simulink library "mylib"  (R2020a)
settings: Solver=VariableStepAuto  StartTime=0.0  StopTime=10.0  RelTol=1e-3
undefined symbols (not defined in the file): d_du_max_pu, dir_to_bus1, dir_to_bus_0L, dir_to_bus_2, dir_to_line1, dir_to_line_0L, dir_to_line_2, du_max_pu, du_ph_max_pu, Fi_0, Fi_T_H, Fi_T_L, Fi_T_M, I0_calc_0L, I0_comp_H, I0_comp_L, I0_comp_M, I0_max_0L, I2_max_2, I_diff1, I_diff2, I_diff3, I_diff4, I_diff5, I_diff_to, I_hight_CT1_G, I_hight_CT2_G, I_low_CT1, I_low_CT2, I_max1, I_max2, I_max3, I_max4, I_max5, I_min_sec_CT1, I_min_sec_CT2, I_unb, Iph_max_0L, Iph_max_2, jmp_in_zone, jmp_in_zone_0L, jmp_in_zone_2, K_dop, max_min1, only_K1_0L, only_K1_2, only_K2_0L, only_K2_2, only_K3_0L, only_K3_2, P_ctl_0, PQ_Fi_ctl_0, Q_ctl_0, S_set_0, set, set1, T_fast, T_I_ctl, T_off, T_on ... (+15)
libraries: $bdroot x184, powerlib_meascontrol x97
(part 1 of 14)
settings Model: Creator=Fasedus  LastModifiedBy=Александр
settings DataIOCC: ReturnWorkspaceOutputs=off
settings DebuggingCC: ArithmeticOperatorsInVariantConditions=warning
settings SFSimCC: SimUseLocalCustomCode=off  CustomCodeUndefinedFunction=UseInterfaceOnly
settings RTWCC: RTWUseLocalCustomCode=off
settings CodeAppCC: StateflowObjectComments=on

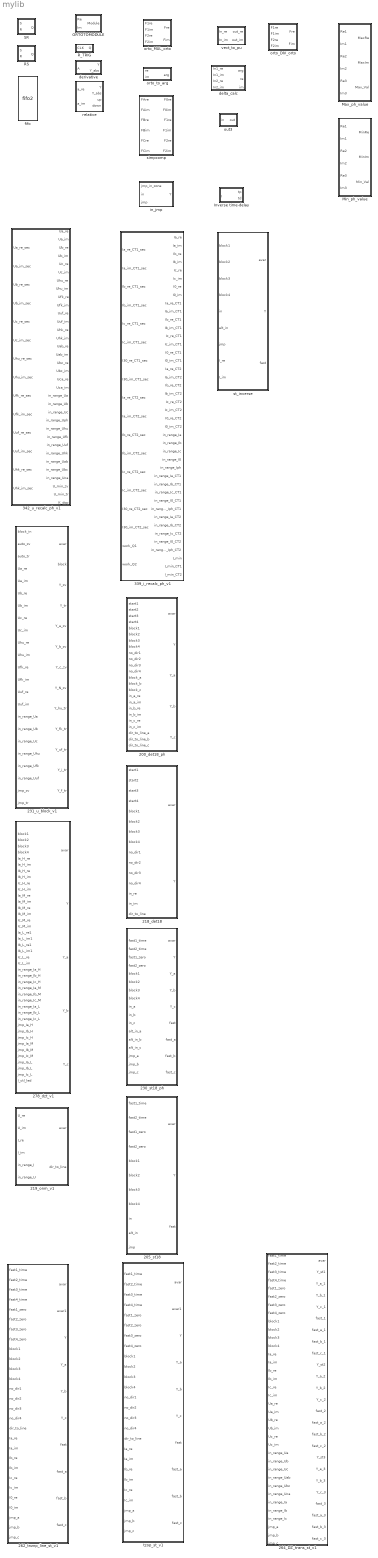
== system mylib ==
  200_det18_ph : Subsystem  mask{det=[max_min1, set1, dir_to_line1, dir_to_bus1]}
      mask prompts: det "det [max_min, set, dir_to_line, dir_to_bus]"
      mask init:
      | max_min = det(1);
      | set = det(2);
      | dir_to_line = det(3);
      | dir_to_bus = det(4);
  205_st18 : Subsystem  AncestorBlock=mylib/205_st18  mask{st18_ph=[1, 1, 1, 0, T_reset, 0, T_st_sign, T_out]}
      mask prompts: st18_ph "st18_ph [only_K1, only_K2, only_K3, jmp_in_zone, T_reset, T_fast, T_st, T_out]"
      mask init:
      | only_K1 = st18_ph(1);
      | only_K2 = st18_ph(2); 
      | only_K3 = st18_ph(3); 
      | jmp_in_zone = st18_ph(4);
      | T_reset = st18_ph(5);
      | T_fast = st18_ph(6); 
      | T_st = st18_ph(7); 
      | T_out = st18_ph(8);
  218_det18 : Subsystem  AncestorBlock=mylib/218_det18  mask{det=[0, set, 0, 0]}
      mask prompts: det "det [max_min, set, dir_to_line, dir_to_bus]"
      mask init:
      | max_min = det(1);
      | set = det(2);
      | dir_to_line = det(3);
      | dir_to_bus = det(4);
  219_onm_v1 : Subsystem  mask{onm_v1=[PQ_Fi_ctl_0, P_ctl_0, Q_ctl_0, U_dir_PQ_0,S_set_0, Fi_0]}
      mask prompts: onm_v1 "onm_v1[PQ_Fi_ctl, P_ctl, Q_ctl, U_dir_PQ,S_set, Fi]"
      mask init:
      | PQ_Fi_ctl= onm_v1(1);
      | P_ctl = onm_v1(2);
      | Q_ctl = onm_v1(3); 
      | U_dir_PQ = onm_v1(4);
      | S_set = onm_v1(5); 
      | Fi = onm_v1(6);
  230_st18_ph : Subsystem  AncestorBlock=mylib/230_st18_ph  mask{st18_ph=[1, 1, 1, 0, T_reset, T_fast, T_st, T_out]}
      mask prompts: st18_ph "st18_ph [only_K1, only_K2, only_K3, jmp_in_zone, T_reset, T_fast, T_st, T_out]"
      mask init:
      | only_K1 = st18_ph(1);
      | only_K2 = st18_ph(2); 
      | only_K3 = st18_ph(3); 
      | jmp_in_zone = st18_ph(4);
      | T_reset = st18_ph(5);
      | T_fast = st18_ph(6); 
      | T_st = st18_ph(7); 
      | T_out = st18_ph(8);
  231_u_block_v1 : Subsystem  mask{Ublock=[K_dop, du_ph_max_pu, du_max_pu, d_du_max_pu]}
      mask prompts: Ublock "Ublock [ K_dop, du_ph_max_pu,du_max_pu, d_du_max_pu]"
      mask init:
      | K_dop = Ublock(1);
      | du_ph_max_pu = Ublock(2);
      | du_max_pu = Ublock(3); 
      | d_du_max_pu = Ublock(4);
  262_tnznp_line_st_v1 : Subsystem  mask{tnznp_line=[I0_calc_0L,I0_max_0L, Iph_max_0L, dir_to_line_0L, dir_to_bus_0L, only_K1_0L, only_K2_0L, only_K3_0L, jmp_in_zone_0L, T_st_0L]}
      mask prompts: tnznp_line "tnznp_line [I0_calc, Iph_max, dir_to_line, dir_to_bus, only_K1, only_K2, only_K3, jmp_in_zone, T_st]"
      mask init:
      | I0_calc = tnznp_line(1);
      | I0_max = tnznp_line(2);
      | Iph_max = tnznp_line(3); 
      | dir_to_line = tnznp_line(4);
      | dir_to_bus = tnznp_line(5);
      | only_K1 = tnznp_line(6); 
      | only_K2 = tnznp_line(7); 
      | only_K3 = tnznp_line(8); 
      | jmp_in_zone = tnznp_line(9); 
      | T_st = tnznp_line(10);
  264_DZ_trans_st_v1 : Subsystem  mask{DZ_trans_time=[1, 2, 3], DZ_trans_Calc1=[5, 0.00151, 0.219, 1000], DZ_trans_Calc2=[0, 20000, 0, 0], DZ_trans_PolySet1=[0, 0, -10, 10, -15, 30, -20, 120, 10, 80, 20, 100], DZ_trans_PolySet2=[40, 100, 40, 70, 60, 70, 80, 40, 90, 30, 20, 30]}
      mask prompts: DZ_trans_time "[T_st1, T_st2, T_st3]"; DZ_trans_Calc1 "[arg_U_K2, R, X, U_kz_pu_r_rem ]"; DZ_trans_Calc2 "[ph_to_line, U_nom_ph, recalc_Z_ph, recalc_Z_lin]"; DZ_trans_PolySet1 "[R_1, X_1, R_2, X_2, R_3, X_3, R_4, X_4, R_5, X_5, R_6, X_6]"; DZ_trans_PolySet2 "[R_7, X_7, R_8, X_8, R_9, X_9, R_10, X_10, R_11, X_11, R_12, X_12]"
      mask init:
      | T_st1 = DZ_trans_time(1);
      | T_st2 = DZ_trans_time(2); 
      | T_st3 = DZ_trans_time(3);
      | 
      | arg_U_K2 = DZ_trans_Calc1(1); 
      | R = DZ_trans_Calc1(2);
      | X = DZ_trans_Calc1(3); 
      | U_kz_pu_r_rem = DZ_trans_Calc1(4);
      | 
      | ph_to_line = DZ_trans_Calc2(1); 
      | U_nom_ph = DZ_trans_Calc2(2);  
      | recalc_Z_ph = DZ_trans_Calc2(3); 
      | recalc_Z_lin = DZ_trans_Calc2(4); 
      | 
      | R_1 = DZ_trans_PolySet1 (1); 
      | X_1 = DZ_trans_PolySet1 (2); 
      | R_2 = DZ_trans_PolySet1 (3); 
      | X_2 = DZ_trans_PolySet1 (4); 
      | R_3 = DZ_trans_PolySet1 (5); 
      | X_3 = DZ_trans_PolySet1 (6); 
      | R_4 = DZ_trans_PolySet1 (7); 
      | X_4 = DZ_trans_PolySet1 (8); 
      | R_5 = DZ_trans_PolySet1 (9); 
      | X_5 = DZ_trans_PolySet1 (10); 
      | R_6 = DZ_trans_PolySet1 (11); 
      | X_6 = DZ_trans_PolySet1 (12);
      | 
      | R_7 = DZ_trans_PolySet2 (1); 
      | X_7 = DZ_trans_PolySet2 (2); 
      | R_8 = DZ_trans_PolySet2 (3); 
      | X_8 = DZ_trans_PolySet2 (4); 
      | R_9 = DZ_trans_PolySet2 (5); 
      | X_9 = DZ_trans_PolySet2 (6); 
      | R_10 = DZ_trans_PolySet2 (7); 
      | X_10 = DZ_trans_PolySet2 (8); 
      | R_11 = DZ_trans_PolySet2 (9); 
      | X_11 = DZ_trans_PolySet2 (10); 
      | R_12 = DZ_trans_PolySet2 (11); 
      | X_12 = DZ_trans_PolySet2 (12);
  278_dzt_v1 : Subsystem  AncestorBlock=mylib/278_dzt_v1  mask{dzt1=[I0_comp_H,I0_comp_M,I0_comp_L], dzt2=[Fi_T_H,Fi_T_M,Fi_T_L], dzt3=[U_H_T,U_M_T,U_L_T], dzt4=[I_diff_to, I_unb, jmp_in_zone], dzt5=[T_I_ctl, T_reset, T_out], dzt6=[I_diff1, I_max1, I_diff2, I_max2, I_diff3, I_max3, I_diff4, I_max4, I_diff5, I_max5]}
      mask prompts: dzt1 "dzt1 [I0_comp_H, I0_comp_M, I0_comp_L]"; dzt2 "dzt2 [Fi_T_H, Fi_T_M, Fi_T_L]"; dzt3 "dzt3[U_H_T, U_M_T, U_L_T]"; dzt4 "dzt4[I_diff_to, I_unb, jmp_in_zone]"; dzt5 "dzt5 [ T_I_ctl, T_reset, T_out]"; dzt6 "dzt6 [I_diff1, I_max1, I_diff2, I_max2, I_diff3, I_max3, I_diff4, I_max4, I_diff5, I_max5]"
      mask init:
      | I0_comp_H = dzt1(1);
      | I0_comp_M = dzt1(2);
      | I0_comp_L = dzt1(3);
      | 
      | Fi_T_H = dzt2(1);
      | Fi_T_M = dzt2(2);
      | Fi_T_L = dzt2(3);
      | 
      | U_H_T = dzt3(1);
      | U_M_T = dzt3(2);
      | U_L_T = dzt3(3);
      | 
      | I_diff_to = dzt4(1);
      | I_unb = dzt4(2);
      | jmp_in_zone = dzt4(3);
      | 
      | T_I_ctl = dzt5(1);
      | T_reset = dzt5(2);
      | T_out = dzt5(3);
      | 
      | I_diff1 = dzt6(1);
      | I_max1 = dzt6(2);
      | I_diff2 = dzt6(3);
      | I_max2 = dzt6(4);
      | I_diff3 = dzt6(5);
      | I_max3 = dzt6(6);
      | I_diff4 = dzt6(7);
      | I_max4 = dzt6(8);
      | I_diff5 = dzt6(9);
      | I_max5 = dzt6(10);
  339_i_recalc_ph_v1 : Subsystem  mask{K_CT=[I_hight_CT1_G, I_low_CT1, I_hight_CT2_G, I_low_CT2], T=[T_on,T_off], I_min=[I_min_sec_CT1, I_min_sec_CT2]}
      mask prompts: K_CT "K_CT [ I_hight_CT1,  I_low_CT1, I_hight_CT2,  I_low_CT2]"; T "T [T_on, T_off]"; I_min "I_min [I_min_sec_CT1,I_min_sec_CT2 ]"
      mask init:
      | I_hight_CT1 = K_CT(1);
      | I_low_CT1 = K_CT(2);
      | I_hight_CT2 = K_CT(3);
      | I_low_CT2 = K_CT(4);
      | 
      | T_on = T(1);
      | T_off = T(2);
      | 
      | 
      | I_min_sec_CT1 = I_min (1);
      | I_min_sec_CT2 = I_min (2);
  342_u_recalc_ph_v1 : Subsystem  mask{K_VT=[U_hight_VT_G, U_low_VT_zv, U_low_VT_tr], U_min=[U_min_sec_zv, U_min_sec_tr]}
      mask prompts: K_VT "K_VT [ U_hight_VT, U_low_VT_zv,U_low_VT_tr]"; U_min "U_min [U_min_sec_zv,U_min_sec_tr ]"
      mask init:
      | U_hight_VT = K_VT(1);
      | U_low_VT_zv = K_VT(2);
      | U_low_VT_tr = K_VT(3);
      | 
      | U_min_sec_zv = U_min (1);
      | U_min_sec_tr = U_min (2);
  Inverse time-delay : Subsystem  mask{Itd=[14.7, 1, 1], IEC=[4, 3, 9, 0.05], IEC_idr=[4, 7, 2], ANSI=[7, 3, 7, 9.3, 0.08], ANSI_idr=[7, 5, 4.1, 0]}
      mask prompts: Itd "Itd [Ip, Type_ITD, IDR]"; IEC "IEC [IEC_N, ku_IEC, au_IEC, Tb]"; IEC_idr "IEC_idr [IEC_N_idr, ku_IEC_idr, au_IEC_idr]"; ANSI "ANSI [ANSI_N, Au_ANSI, Bu_ANSI, Cu_ANSI, D]"; ANSI_idr "ANSI_idr [ANSI_N_idr, Au_ANSI_idr, Bu_ANSI_idr, Cu_ANSI_idr]"
      mask init:
      | Ip = Itd (1);
      | Type_ITD = Itd (2);
      | IDR = Itd (3);
      | 
      | IEC_N = IEC(1); 
      | ku_IEC = IEC(2); 
      | au_IEC = IEC(3);
      | Tb = IEC(4);
      | 
      | IEC_N_idr = IEC_idr(1); 
      | ku_IEC_idr = IEC_idr(2);
      | au_IEC_idr = IEC_idr(3);
      | 
      | ANSI_N = ANSI(1); 
      | Au_ANSI = ANSI(2);
      | Bu_ANSI = ANSI(3); 
      | Cu_ANSI = ANSI(4); 
      | D = ANSI(5);
      | 
      | ANSI_N_idr = ANSI_idr(1); 
      | Au_ANSI_idr = ANSI_idr(2);
      | Bu_ANSI_idr = ANSI_idr(3); 
      | Cu_ANSI_idr = ANSI_idr(4);
      mask DialogControl Control2 Prompt: Inverse time-delay
      mask DialogControl Control3 Prompt: IEC
      mask DialogControl Control4 Prompt: IEC_idr
      mask DialogControl Control5 Prompt: ANSI
      mask DialogControl Control6 Prompt: ANSI_idr
  Max_ph_value : Subsystem
  Min_ph_value : Subsystem
  ORTOTOMODULE : Subsystem
  RS : Subsystem
  R_TRIG : Subsystem
  SR : Subsystem
  delta_calc : Subsystem
  derivative : Subsystem
  fifo : $bdroot/relative/fifo2  SystemSampleTime=-1  Latency=0  AutoFrameSizeCalculation=off
  in_jmp : Subsystem  mask{in_jmp=[T_reset]}
      mask prompts: in_jmp "in_jmp[T_reset]"
  orto_DIV_orto : Subsystem  AncestorBlock=mylib/orto_MUL_orto
  orto_MUL_orto : Subsystem
  orto_to_arg : Subsystem
  out3 : Subsystem  mask{out=[T_out]}
      mask prompts: out "out[T_out]"
      mask init:
      | T_out = out(1);
  relative : Subsystem
  simpcomp : Subsystem
  st_inverse : Subsystem  AncestorBlock=mylib/205_st18  mask{st18_ph=[1, 1, 1, 0, T_reset, T_fast, T_st, T_out], Itd=[14.7, 1, 1], IEC=[4, 3, 9, 0.05], IEC_idr=[4, 7, 2], ANSI=[7, 3, 7, 9.3, 0.08], ANSI_idr=[7, 5, 4.1, 0]}
      mask prompts: st18_ph "st18_ph [only_K1, only_K2, only_K3, jmp_in_zone, T_reset, T_fast, T_st, T_out]"; Itd "Itd [Ip, Type_ITD, IDR]"; IEC "IEC [IEC_N, ku_IEC, au_IEC, Tb]"; IEC_idr "IEC_idr [IEC_N_idr, ku_IEC_idr, au_IEC_idr]"; ANSI "ANSI [ANSI_N, Au_ANSI, Bu_ANSI, Cu_ANSI, D]"; ANSI_idr "ANSI_idr [ANSI_N_idr, Au_ANSI_idr, Bu_ANSI_idr, Cu_ANSI_idr]"
      mask init:
      | only_K1 = st18_ph(1);
      | only_K2 = st18_ph(2); 
      | only_K3 = st18_ph(3); 
      | jmp_in_zone = st18_ph(4);
      | T_reset = st18_ph(5);
      | T_fast = st18_ph(6); 
      | T_st = st18_ph(7); 
      | T_out = st18_ph(8);
      | 
      | Ip = Itd (1);
      | Type_ITD = Itd (2);
      | IDR = Itd (3);
      | 
      | IEC_N = IEC(1); 
      | ku_IEC = IEC(2); 
      | au_IEC = IEC(3);
      | Tb = IEC(4);
      | 
      | IEC_N_idr = IEC_idr(1); 
      | ku_IEC_idr = IEC_idr(2);
      | au_IEC_idr = IEC_idr(3);
      | 
      | ANSI_N = ANSI(1); 
      | Au_ANSI = ANSI(2);
      | Bu_ANSI = ANSI(3); 
      | Cu_ANSI = ANSI(4); 
      | D = ANSI(5);
      | 
      | ANSI_N_idr = ANSI_idr(1); 
      | Au_ANSI_idr = ANSI_idr(2);
      | Bu_ANSI_idr = ANSI_idr(3); 
      | Cu_ANSI_idr = ANSI_idr(4);
      mask DialogControl Control2 Prompt: Inverse time-delay
      mask DialogControl Control3 Prompt: IEC
      mask DialogControl Control4 Prompt: IEC_idr
      mask DialogControl Control5 Prompt: ANSI
      mask DialogControl Control6 Prompt: ANSI_idr
  tzop_st_v1 : Subsystem  mask{tzop=[I2_max_2, Iph_max_2, dir_to_line_2, dir_to_bus_2, only_K1_2, only_K2_2, only_K3_2, jmp_in_zone_2, T_st_2]}
      mask prompts: tzop "tzop [I2_max,Iph_max, dir_to_line, dir_to_bus, only_K1, only_K2, only_K3, jmp_in_zone, T_st]"
      mask init:
      | I2_max = tzop(1);
      | Iph_max = tzop(2); 
      | dir_to_line = tzop(3);
      | dir_to_bus = tzop(4);
      | only_K1 = tzop(5); 
      | only_K2 = tzop(6); 
      | only_K3 = tzop(7); 
      | jmp_in_zone = tzop(8); 
      | T_st = tzop(9);
  vect_to_pu : Subsystem

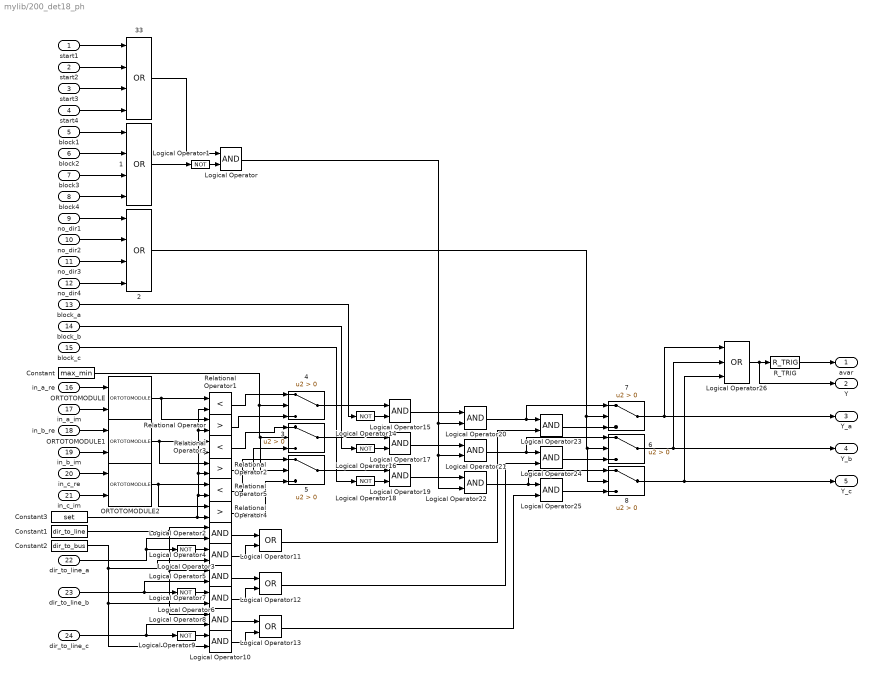
== system mylib/200_det18_ph ==
  start1 : Inport
  start2 : Inport  Port=2
  start3 : Inport  Port=3
  start4 : Inport  Port=4
  block1 : Inport  Port=5
  block2 : Inport  Port=6
  block3 : Inport  Port=7
  block4 : Inport  Port=8
  no_dir1 : Inport  Port=9
  no_dir2 : Inport  Port=10
  no_dir3 : Inport  Port=11
  no_dir4 : Inport  Port=12
  block_a : Inport  Port=13
  block_b : Inport  Port=14
  block_c : Inport  Port=15
  in_a_re : Inport  Port=16
  in_a_im : Inport  Port=17
  in_b_re : Inport  Port=18
  in_b_im : Inport  Port=19
  in_c_re : Inport  Port=20
  in_c_im : Inport  Port=21
  dir_to_line_a : Inport  Port=22
  dir_to_line_b : Inport  Port=23
  dir_to_line_c : Inport  Port=24
  1 : Logic  Operator=OR  Inputs=4  AllPortsSameDT=off  OutDataTypeStr=boolean
  2 : Logic  Operator=OR  Inputs=4  AllPortsSameDT=off  OutDataTypeStr=boolean
  {3..8} (6 alike) : Switch  Criteria=u2 > Threshold
  33 : Logic  Operator=OR  Inputs=4  AllPortsSameDT=off  OutDataTypeStr=boolean
  Constant : Constant  Value=max_min
  Constant1 : Constant  Value=dir_to_line
  Constant2 : Constant  Value=dir_to_bus
  Constant3 : Constant  Value=set
  Logical Operator{,2,4..5,7..8,10,15,17,19..25} (16 alike) : Logic  AllPortsSameDT=off  OutDataTypeStr=boolean
  Logical Operator{1,3,6,9,14,16,18} (7 alike) : Logic  Operator=NOT  AllPortsSameDT=off  OutDataTypeStr=boolean
  Logical Operator11 : Logic  Operator=OR  AllPortsSameDT=off  OutDataTypeStr=boolean
  Logical Operator12 : Logic  Operator=OR  AllPortsSameDT=off  OutDataTypeStr=boolean
  Logical Operator13 : Logic  Operator=OR  AllPortsSameDT=off  OutDataTypeStr=boolean
  Logical Operator26 : Logic  Operator=OR  Inputs=3  AllPortsSameDT=off  OutDataTypeStr=boolean
  ORTOTOMODULE : $bdroot/ORTOTOMODULE  SystemSampleTime=-1  Latency=0  AutoFrameSizeCalculation=off
  ORTOTOMODULE1 : $bdroot/ORTOTOMODULE  SystemSampleTime=-1  Latency=0  AutoFrameSizeCalculation=off
  ORTOTOMODULE2 : $bdroot/ORTOTOMODULE  SystemSampleTime=-1  Latency=0  AutoFrameSizeCalculation=off
  R_TRIG : $bdroot/R_TRIG  SystemSampleTime=-1  Latency=0  AutoFrameSizeCalculation=off
  Relational Operator : RelationalOperator  Operator=>  OutDataTypeStr=boolean  RndMeth=Simplest
  Relational Operator1 : RelationalOperator  Operator=<  OutDataTypeStr=boolean  RndMeth=Simplest
  Relational Operator2 : RelationalOperator  Operator=>  OutDataTypeStr=boolean  RndMeth=Simplest
  Relational Operator3 : RelationalOperator  Operator=<  OutDataTypeStr=boolean  RndMeth=Simplest
  Relational Operator4 : RelationalOperator  Operator=>  OutDataTypeStr=boolean  RndMeth=Simplest
  Relational Operator5 : RelationalOperator  Operator=<  OutDataTypeStr=boolean  RndMeth=Simplest
  avar : Outport
  Y : Outport  Port=2
  Y_a : Outport  Port=3
  Y_b : Outport  Port=4
  Y_c : Outport  Port=5
  wires:
  start1/1 -> 33/1
  start4/1 -> 33/4
  start3/1 -> 33/3
  start2/1 -> 33/2
  block1/1 -> 1/1
  block2/1 -> 1/2
  block3/1 -> 1/3
  block4/1 -> 1/4
  no_dir1/1 -> 2/1
  no_dir2/1 -> 2/2
  no_dir3/1 -> 2/3
  no_dir4/1 -> 2/4
  Logical Operator1/1 -> Logical Operator/2
  1/1 -> Logical Operator1/1
  33/1 -> Logical Operator/1
  in_a_im/1 -> ORTOTOMODULE/2
  in_a_re/1 -> ORTOTOMODULE/1
  ORTOTOMODULE/1 -> Relational Operator1/1, Relational Operator/1
  ORTOTOMODULE1/1 -> Relational Operator2/1, Relational Operator3/1
  in_b_im/1 -> ORTOTOMODULE1/2
  ORTOTOMODULE2/1 -> Relational Operator5/1, Relational Operator4/1
  in_c_im/1 -> ORTOTOMODULE2/2
  in_c_re/1 -> ORTOTOMODULE2/1
  Constant/1 -> 5/2, 3/2, 4/2
  Relational Operator/1 -> 4/3
  Relational Operator2/1 -> 3/3
  Relational Operator4/1 -> 5/3
  Relational Operator5/1 -> 5/1
  Relational Operator3/1 -> 3/1
  Constant3/1 -> Relational Operator2/2, Relational Operator1/2, Relational Operator/2, Relational Operator3/2, Relational Operator5/2, Relational Operator4/2
  Relational Operator1/1 -> 4/1
  Constant1/1 -> Logical Operator2/1, Logical Operator8/1, Logical Operator5/1
  dir_to_line_a/1 -> Logical Operator2/2, Logical Operator3/1
  Logical Operator3/1 -> Logical Operator4/1
  Logical Operator6/1 -> Logical Operator7/1
  Logical Operator9/1 -> Logical Operator10/1
  dir_to_line_b/1 -> Logical Operator5/2, Logical Operator6/1
  dir_to_line_c/1 -> Logical Operator8/2, Logical Operator9/1
  Constant2/1 -> Logical Operator4/2, Logical Operator7/2, Logical Operator10/2
  Logical Operator2/1 -> Logical Operator11/1
  Logical Operator4/1 -> Logical Operator11/2
  Logical Operator5/1 -> Logical Operator12/1
  Logical Operator7/1 -> Logical Operator12/2
  Logical Operator8/1 -> Logical Operator13/1
  Logical Operator10/1 -> Logical Operator13/2
  Logical Operator14/1 -> Logical Operator15/2
  4/1 -> Logical Operator15/1
  Logical Operator16/1 -> Logical Operator17/2
  3/1 -> Logical Operator17/1
  Logical Operator18/1 -> Logical Operator19/2
  5/1 -> Logical Operator19/1
  block_c/1 -> Logical Operator18/1
  block_b/1 -> Logical Operator16/1
  block_a/1 -> Logical Operator14/1
  Logical Operator15/1 -> Logical Operator20/1
  Logical Operator17/1 -> Logical Operator21/1
  Logical Operator19/1 -> Logical Operator22/1
  Logical Operator/1 -> Logical Operator20/2, Logical Operator21/2, Logical Operator22/2
  Logical Operator20/1 -> 7/1, Logical Operator23/1
  Logical Operator21/1 -> 6/1, Logical Operator24/1
  Logical Operator22/1 -> 8/1, Logical Operator25/1
  Logical Operator11/1 -> Logical Operator23/2
  Logical Operator12/1 -> Logical Operator24/2
  2/1 -> 8/2, 6/2, 7/2
  Logical Operator13/1 -> Logical Operator25/2
  Logical Operator24/1 -> 6/3
  Logical Operator23/1 -> 7/3
  Logical Operator25/1 -> 8/3
  8/1 -> Y_c/1, Logical Operator26/3
  6/1 -> Y_b/1, Logical Operator26/2
  7/1 -> Y_a/1, Logical Operator26/1
  Logical Operator26/1 -> Y/1, R_TRIG/1
  R_TRIG/1 -> avar/1
  in_b_re/1 -> ORTOTOMODULE1/1

== system mylib/205_st18 ==
  fast1_time : Inport
  fast2_time : Inport  Port=2
  fast1_zero : Inport  Port=3
  fast2_zero : Inport  Port=4
  block1 : Inport  Port=5
  block2 : Inport  Port=6
  block3 : Inport  Port=7
  block4 : Inport  Port=8
  in : Inport  Port=9
  alt_in : Inport  Port=10
  jmp : Inport  Port=11
  1 : Logic  Operator=OR  Inputs=4  AllPortsSameDT=off  OutDataTypeStr=boolean
  Constant4 : Constant  Value=jmp_in_zone
  Logical Operator14 : Logic  Operator=OR  AllPortsSameDT=off  OutDataTypeStr=boolean
  Logical Operator2 : Logic  AllPortsSameDT=off  OutDataTypeStr=boolean
  Logical Operator27 : Logic  Operator=OR  AllPortsSameDT=off  OutDataTypeStr=boolean
  Logical Operator28 : Logic  Operator=OR  AllPortsSameDT=off  OutDataTypeStr=boolean
  Logical Operator3 : Logic  Operator=NOT  AllPortsSameDT=off  OutDataTypeStr=boolean
  Logical Operator8 : Logic  AllPortsSameDT=off  OutDataTypeStr=boolean
  R_TRIG : $bdroot/R_TRIG  SystemSampleTime=-1  Latency=0  AutoFrameSizeCalculation=off
  Subsystem : Subsystem  mask{time=[T_fast, T_st]}
      mask prompts: time "time [T_fast, T_st]"
  in_1 : Subsystem  mask{in_jmp=[T_reset]}
      mask prompts: in_jmp "in_jmp[T_reset]"
  out_a : $bdroot/out3  out=[T_out]
  avar : Outport
  Y : Outport  Port=2
  fast : Outport  Port=3
  wires:
  fast1_time/1 -> Logical Operator27/1
  fast2_zero/1 -> Logical Operator28/2
  fast1_zero/1 -> Logical Operator28/1
  fast2_time/1 -> Logical Operator27/2
  block1/1 -> 1/1
  block2/1 -> 1/2
  block3/1 -> 1/3
  block4/1 -> 1/4
  in/1 -> Logical Operator8/2, in_1/2(in)
  R_TRIG/1 -> avar/1
  Constant4/1 -> in_1/1(jmp_in_zone)
  jmp/1 -> in_1/3(jmp)
  Logical Operator3/1 -> Logical Operator2/1
  in_1/1(Y) -> Logical Operator2/2  "Ya"
  1/1 -> Logical Operator3/1
  out_a/1 -> Y/1, R_TRIG/1  "Y_c"
  Logical Operator8/1 -> out_a/1
  Subsystem/1(Out1) -> Logical Operator8/1
  Logical Operator2/1 -> fast/1, Logical Operator14/1
  Logical Operator14/1 -> Subsystem/3("In1 ")
  alt_in/1 -> Logical Operator14/2
  Logical Operator27/1 -> Subsystem/1(T_fast_time)
  Logical Operator28/1 -> Subsystem/2(T_fast_zero)

== system mylib/218_det18 ==
  start1 : Inport
  start2 : Inport  Port=2
  start3 : Inport  Port=3
  start4 : Inport  Port=4
  block1 : Inport  Port=5
  block2 : Inport  Port=6
  block3 : Inport  Port=7
  block4 : Inport  Port=8
  no_dir1 : Inport  Port=9
  no_dir2 : Inport  Port=10
  no_dir3 : Inport  Port=11
  no_dir4 : Inport  Port=12
  in_re : Inport  Port=13
  in_im : Inport  Port=14
  dir_to_line : Inport  Port=15
  1 : Logic  Operator=OR  Inputs=4  AllPortsSameDT=off  OutDataTypeStr=boolean
  2 : Logic  Operator=OR  Inputs=4  AllPortsSameDT=off  OutDataTypeStr=boolean
  33 : Logic  Operator=OR  Inputs=4  AllPortsSameDT=off  OutDataTypeStr=boolean
  4 : Switch  Criteria=u2 > Threshold
  7 : Switch  Criteria=u2 > Threshold
  Constant : Constant  Value=max_min
  Constant1 : Constant  Value=dir_to_line
  Constant2 : Constant  Value=dir_to_bus
  Constant3 : Constant  Value=set
  Logical Operator{,2,4,20,23} (5 alike) : Logic  AllPortsSameDT=off  OutDataTypeStr=boolean
  Logical Operator1 : Logic  Operator=NOT  AllPortsSameDT=off  OutDataTypeStr=boolean
  Logical Operator11 : Logic  Operator=OR  AllPortsSameDT=off  OutDataTypeStr=boolean
  Logical Operator3 : Logic  Operator=NOT  AllPortsSameDT=off  OutDataTypeStr=boolean
  ORTOTOMODULE : $bdroot/ORTOTOMODULE  SystemSampleTime=-1  Latency=0  AutoFrameSizeCalculation=off
  R_TRIG : $bdroot/R_TRIG  SystemSampleTime=-1  Latency=0  AutoFrameSizeCalculation=off
  Relational Operator : RelationalOperator  Operator=>  OutDataTypeStr=boolean  RndMeth=Simplest
  Relational Operator1 : RelationalOperator  Operator=<  OutDataTypeStr=boolean  RndMeth=Simplest
  Scope : Scope
  avar : Outport
  Y : Outport  Port=2
  wires:
  start1/1 -> 33/1
  start4/1 -> 33/4
  start3/1 -> 33/3
  start2/1 -> 33/2
  block1/1 -> 1/1
  block2/1 -> 1/2
  block3/1 -> 1/3
  block4/1 -> 1/4
  no_dir1/1 -> 2/1
  no_dir2/1 -> 2/2
  no_dir3/1 -> 2/3
  no_dir4/1 -> 2/4
  Logical Operator1/1 -> Logical Operator/2
  1/1 -> Logical Operator1/1
  33/1 -> Logical Operator/1
  in_im/1 -> ORTOTOMODULE/2
  in_re/1 -> ORTOTOMODULE/1
  ORTOTOMODULE/1 -> Scope/1, Relational Operator1/1, Relational Operator/1
  Constant/1 -> 4/2
  Relational Operator/1 -> 4/3
  Constant3/1 -> Relational Operator1/2, Relational Operator/2
  Relational Operator1/1 -> 4/1
  Constant1/1 -> Logical Operator2/1
  dir_to_line/1 -> Logical Operator2/2, Logical Operator3/1
  Logical Operator3/1 -> Logical Operator4/2
  Constant2/1 -> Logical Operator4/1
  Logical Operator2/1 -> Logical Operator11/1
  Logical Operator4/1 -> Logical Operator11/2
  4/1 -> Logical Operator20/1
  Logical Operator/1 -> Logical Operator20/2
  Logical Operator20/1 -> 7/1, Logical Operator23/1
  Logical Operator11/1 -> Logical Operator23/2
  2/1 -> 7/2
  Logical Operator23/1 -> 7/3
  7/1 -> Y/1, R_TRIG/1
  R_TRIG/1 -> avar/1

== system mylib/219_onm_v1 ==
  U_re : Inport
  U_im : Inport  Port=2
  I_re : Inport  Port=3
  I_im : Inport  Port=4
  in_range_I : Inport  Port=5
  in_range_U : Inport  Port=6
  Constant : Constant  Value=0
  Constant1 : Constant
  Constant2 : Constant  Value=U_dir_PQ
  Constant3 : Constant  Value=PQ_Fi_ctl
  Logical Operator : Logic  Operator=NOT  AllPortsSameDT=off  OutDataTypeStr=boolean
  Logical Operator1 : Logic  Operator=OR  AllPortsSameDT=off  OutDataTypeStr=boolean
  Logical Operator2 : Logic  Operator=NOT  AllPortsSameDT=off  OutDataTypeStr=boolean
  ORTOTOMODULE : $bdroot/ORTOTOMODULE  SystemSampleTime=-1  Latency=0  AutoFrameSizeCalculation=off
  Relational Operator : RelationalOperator  Operator=<  OutDataTypeStr=boolean  RndMeth=Simplest
  Switch : Switch  Criteria=u2 > Threshold
  Switch1 : Switch  Criteria=u2 > Threshold
  onm_fi_v1 : Subsystem  mask{onm_fi_v1=[S_set, Fi]}
      mask prompts: onm_fi_v1 "onm_fi_v1[S_set, Fi]"
      mask init:
      | S_set = onm_fi_v1(1);
      | Fi = onm_fi_v1(2);
      mask DialogControl Control2 Prompt: onm_fi_v1
  pq_dir_v1 : Subsystem  mask{pq_dir_v1=[P_ctl, Q_ctl]}
      mask prompts: pq_dir_v1 "pq_dir_v1[P_ctl, Q_ctl]"
      mask init:
      | P_ctl = pq_dir_v1(1);
      | Q_ctl = pq_dir_v1(2);
      mask DialogControl Control2 Prompt: pq_dir_v1
  avar : Outport
  dir_to_line : Outport  Port=2
  wires:
  in_range_U/1 -> Logical Operator2/1
  in_range_I/1 -> Logical Operator/1
  Constant3/1 -> Switch1/2
  Constant2/1 -> Relational Operator/2
  Relational Operator/1 -> pq_dir_v1/5(max_comp)
  I_im/1 -> pq_dir_v1/4(I_im), onm_fi_v1/4(I_im)
  onm_fi_v1/1(Y) -> Switch1/1
  pq_dir_v1/1(Y) -> Switch1/3
  Switch1/1 -> Switch/3
  Constant1/1 -> Switch/1
  Logical Operator1/1 -> Switch/2
  Logical Operator2/1 -> Logical Operator1/2
  Logical Operator/1 -> Logical Operator1/1
  Switch/1 -> dir_to_line/1
  Constant/1 -> avar/1
  U_im/1 -> ORTOTOMODULE/2, onm_fi_v1/2(U_im), pq_dir_v1/2(U_im)
  U_re/1 -> ORTOTOMODULE/1, onm_fi_v1/1(U_re), pq_dir_v1/1(U_re)
  ORTOTOMODULE/1 -> Relational Operator/1
  I_re/1 -> onm_fi_v1/3(I_re), pq_dir_v1/3(I_re)

== system mylib/230_st18_ph ==
  fast1_time : Inport
  fast2_time : Inport  Port=2
  fast1_zero : Inport  Port=3
  fast2_zero : Inport  Port=4
  block1 : Inport  Port=5
  block2 : Inport  Port=6
  block3 : Inport  Port=7
  block4 : Inport  Port=8
  in_a : Inport  Port=9
  in_b : Inport  Port=10
  in_c : Inport  Port=11
  alt_in_a : Inport  Port=12
  alt_in_b : Inport  Port=13
  alt_in_c : Inport  Port=14
  jmp_a : Inport  Port=15
  jmp_b : Inport  Port=16
  jmp_c : Inport  Port=17
  1 : Logic  Operator=OR  Inputs=4  AllPortsSameDT=off  OutDataTypeStr=boolean
  Constant1 : Constant  Value=only_K2
  Constant2 : Constant  Value=only_K3
  Constant3 : Constant  Value=only_K1
  Constant4 : Constant  Value=jmp_in_zone
  Logical Operator1 : Logic  Operator=OR  Inputs=3  AllPortsSameDT=off  OutDataTypeStr=boolean
  Logical Operator10 : Logic  Inputs=3  AllPortsSameDT=off  OutDataTypeStr=boolean
  Logical Operator{2,4,6,11..13} (6 alike) : Logic  AllPortsSameDT=off  OutDataTypeStr=boolean
  Logical Operator{14,16..17,27..28} (5 alike) : Logic  Operator=OR  AllPortsSameDT=off  OutDataTypeStr=boolean
  Logical Operator26 : Logic  Operator=OR  Inputs=3  AllPortsSameDT=off  OutDataTypeStr=boolean
  Logical Operator3 : Logic  Operator=NOT  AllPortsSameDT=off  OutDataTypeStr=boolean
  Logical Operator5 : Logic  Operator=NOT  AllPortsSameDT=off  OutDataTypeStr=boolean
  Logical Operator7 : Logic  Operator=NOT  AllPortsSameDT=off  OutDataTypeStr=boolean
  Logical Operator8 : Logic  Inputs=3  AllPortsSameDT=off  OutDataTypeStr=boolean
  Logical Operator9 : Logic  Inputs=3  AllPortsSameDT=off  OutDataTypeStr=boolean
  R_TRIG : $bdroot/R_TRIG  SystemSampleTime=-1  Latency=0  AutoFrameSizeCalculation=off
  Subsystem : Subsystem  mask{time=[T_fast, T_st]}
      mask prompts: time "time [T_fast, T_st]"
  in_1 : Subsystem  mask{in_jmp=[T_reset]}
      mask prompts: in_jmp "in_jmp[T_reset]"
  in_2 : Subsystem  mask{in_jmp=[T_reset]}
      mask prompts: in_jmp "in_jmp[T_reset]"
  in_3 : Subsystem  mask{in_jmp=[T_reset]}
      mask prompts: in_jmp "in_jmp[T_reset]"
  k_type : Subsystem
  out_a : $bdroot/out3  out=[T_out]
  out_b : $bdroot/out3  out=[T_out]
  out_c : $bdroot/out3  out=[T_out]
  avar : Outport
  Y : Outport  Port=2
  Y_a : Outport  Port=3
  Y_b : Outport  Port=4
  Y_c : Outport  Port=5
  fast : Outport  Port=6
  fast_a : Outport  Port=7
  fast_b : Outport  Port=8
  fast_c : Outport  Port=9
  wires:
  fast1_time/1 -> Logical Operator27/1
  fast2_zero/1 -> Logical Operator28/2
  fast1_zero/1 -> Logical Operator28/1
  fast2_time/1 -> Logical Operator27/2
  block1/1 -> 1/1
  block2/1 -> 1/2
  block3/1 -> 1/3
  block4/1 -> 1/4
  in_a/1 -> in_1/2(in), Logical Operator8/1
  in_c/1 -> in_3/2(in), Logical Operator10/1
  Logical Operator26/1 -> Y/1, R_TRIG/1
  R_TRIG/1 -> avar/1
  in_b/1 -> in_2/2(in), Logical Operator9/1
  Constant4/1 -> in_3/1(jmp_in_zone), in_2/1(jmp_in_zone), in_1/1(jmp_in_zone)
  jmp_a/1 -> in_1/3(jmp)
  jmp_b/1 -> in_2/3(jmp)
  jmp_c/1 -> in_3/3(jmp)
  Logical Operator3/1 -> Logical Operator2/1
  in_1/1(Y) -> Logical Operator2/2  "Ya"
  Logical Operator5/1 -> Logical Operator4/1
  in_2/1(Y) -> Logical Operator4/2  "Yb"
  Logical Operator7/1 -> Logical Operator6/1
  in_3/1(Y) -> Logical Operator6/2  "Yc"
  1/1 -> Logical Operator7/1, Logical Operator5/1, Logical Operator3/1
  out_a/1 -> Logical Operator26/1, Y_a/1  "Y_c"
  out_b/1 -> Logical Operator26/2, Y_b/1  "Y_c"
  out_c/1 -> Logical Operator26/3, Y_c/1  "Y_c"
  Logical Operator8/1 -> out_a/1
  Logical Operator9/1 -> out_b/1
  Logical Operator10/1 -> out_c/1
  Subsystem/3(Out3) -> Logical Operator10/2
  Subsystem/2(Out2) -> Logical Operator9/2
  Subsystem/1(Out1) -> Logical Operator8/2
  Logical Operator2/1 -> Logical Operator1/1, fast_a/1, Logical Operator11/2, k_type/1(In_a)
  Logical Operator4/1 -> Logical Operator1/2, fast_b/1, Logical Operator12/2, k_type/2(In_b)
  Logical Operator6/1 -> Logical Operator1/3, fast_c/1, Logical Operator13/2, k_type/3(In_ c)
  Constant3/1 -> k_type/4(only_K1)
  Constant1/1 -> k_type/5(only_K2)
  Constant2/1 -> k_type/6(only_K3)
  k_type/1(out) -> Logical Operator10/3, Logical Operator9/3, Logical Operator8/3, Logical Operator12/1, Logical Operator13/1, Logical Operator11/1
  Logical Operator11/1 -> Logical Operator14/1
  Logical Operator12/1 -> Logical Operator16/1
  Logical Operator13/1 -> Logical Operator17/1
  Logical Operator17/1 -> Subsystem/5("In3 ")
  Logical Operator16/1 -> Subsystem/4("In2 ")
  Logical Operator14/1 -> Subsystem/3("In1 ")
  alt_in_a/1 -> Logical Operator14/2
  alt_in_b/1 -> Logical Operator16/2
  alt_in_c/1 -> Logical Operator17/2
  Logical Operator27/1 -> Subsystem/1(T_fast_time)
  Logical Operator28/1 -> Subsystem/2(T_fast_zero)
  Logical Operator1/1 -> fast/1

== system mylib/231_u_block_v1 ==
  block_in : Inport
  auto_zv : Inport  Port=2
  auto_tr : Inport  Port=3
  Ua_re : Inport  Port=4
  Ua_im : Inport  Port=5
  Ub_re : Inport  Port=6
  Ub_im : Inport  Port=7
  Uc_re : Inport  Port=8
  Uc_im : Inport  Port=9
  Uhu_re : Inport  Port=10
  Uhu_im : Inport  Port=11
  Ufk_re : Inport  Port=12
  Ufk_im : Inport  Port=13
  Uuf_re : Inport  Port=14
  Uuf_im : Inport  Port=15
  in_range_Ua : Inport  Port=16
  in_range_Ub : Inport  Port=17
  in_range_Uc : Inport  Port=18
  in_range_Uhu : Inport  Port=19
  in_range_Ufk : Inport  Port=20
  in_range_Uuf : Inport  Port=21
  jmp_zv : Inport  Port=22
  jmp_tr : Inport  Port=23
  1 : Logic  AllPortsSameDT=off  OutDataTypeStr=boolean
  15 : Constant  Value=du_max_pu
  18 : Constant  Value=du_ph_max_pu
  19 : Constant  Value=d_du_max_pu
  2 : Logic  Operator=NOT  AllPortsSameDT=off  OutDataTypeStr=boolean
  20 : Constant  Value=K_dop
  24 : Logic  AllPortsSameDT=off  OutDataTypeStr=boolean
  25 : Logic  Operator=NOT  AllPortsSameDT=off  OutDataTypeStr=boolean
  3 : Logic  Operator=OR  Inputs=3  AllPortsSameDT=off  OutDataTypeStr=boolean
  4 : Logic  Operator=OR  AllPortsSameDT=off  OutDataTypeStr=boolean
  5 : Logic  Operator=OR  AllPortsSameDT=off  OutDataTypeStr=boolean
  6 : Logic  Operator=OR  AllPortsSameDT=off  OutDataTypeStr=boolean
  7 : Logic  Operator=NOT  AllPortsSameDT=off  OutDataTypeStr=boolean
  RS : Subsystem
  U_ctl_calc19 : Subsystem
  U_ctl_logic19 : Subsystem
  oscillo1 : Subsystem
  oscillo2 : Subsystem
  avar : Outport
  block : Outport  Port=2
  Y_zv : Outport  Port=3
  Y_tr : Outport  Port=4
  Y_a_zv : Outport  Port=5
  Y_b_zv : Outport  Port=6
  Y_c_zv : Outport  Port=7
  Y_N_zv : Outport  Port=8
  Y_hu_tr : Outport  Port=9
  Y_fk_tr : Outport  Port=10
  Y_uf_tr : Outport  Port=11
  Y_i_tr : Outport  Port=12
  Y_f_tr : Outport  Port=13
  wires:
  block_in/1 -> 2/1, 24/2
  20/1 -> U_ctl_calc19/19(K_dop)
  18/1 -> U_ctl_calc19/20(du_ph_max_pu)
  15/1 -> U_ctl_calc19/21(du_max_pu)
  19/1 -> U_ctl_calc19/22(d_du_max_pu)
  U_ctl_logic19/1(Y_zv) -> oscillo1/1(CLK), 3/1, Y_zv/1  "Y_zv"
  U_ctl_logic19/2(Y_tr) -> oscillo2/1(CLK), Y_tr/1  "Y_tr"
  U_ctl_logic19/11(Y_f_tr) -> Y_f_tr/1  "Y_f_tr"
  U_ctl_logic19/10(Y_i_tr) -> Y_i_tr/1  "Y_i_tr"
  U_ctl_logic19/9(Y_uf_tr) -> Y_uf_tr/1  "Y_uf_tr"
  U_ctl_logic19/8(Y_fk_tr) -> Y_fk_tr/1  "Y_fk_tr"
  U_ctl_logic19/7(Y_hu_tr) -> Y_hu_tr/1  "Y_hu_tr"
  U_ctl_logic19/6(Y_N_zv) -> Y_N_zv/1  "Y_N_zv"
  U_ctl_logic19/5(Y_c_zv) -> Y_c_zv/1  "Y_c_zv"
  U_ctl_logic19/4(Y_b_zv) -> Y_b_zv/1  "Y_b_zv"
  U_ctl_logic19/3(Y_a_zv) -> Y_a_zv/1  "Y_a_zv"
  25/1 -> 24/1
  2/1 -> 1/1
  24/1 -> 3/3
  3/1 -> RS/1(S)
  6/1 -> RS/2(R)
  RS/1(Q) -> block/1  "block"
  4/1 -> avar/1  "avat"
  oscillo1/1(Q) -> 4/1
  oscillo2/1(Q) -> 4/2
  U_ctl_logic19/12(no_fall) -> 1/2, 25/1
  jmp_zv/1 -> U_ctl_logic19/15(jmp_zv)
  jmp_tr/1 -> U_ctl_logic19/16(jmp_tr)
  in_range_Uuf/1 -> U_ctl_calc19/18(in_range_Uuf)
  in_range_Ufk/1 -> U_ctl_calc19/17(in_range_Ufk)
  in_range_Uhu/1 -> U_ctl_calc19/16(in_range_Uhu)
  in_range_Uc/1 -> U_ctl_calc19/15(in_range_Uc)
  in_range_Ub/1 -> U_ctl_calc19/14(in_range_Ub)
  in_range_Ua/1 -> U_ctl_calc19/13(in_range_Ua)
  Uuf_im/1 -> U_ctl_calc19/12(Uif_im)
  Uuf_re/1 -> U_ctl_calc19/11(Uif_re)
  Ufk_im/1 -> U_ctl_calc19/10(Ufk_im)
  Ufk_re/1 -> U_ctl_calc19/9(Ufk_re)
  Uhu_im/1 -> U_ctl_calc19/8(Uni_im)
  Uhu_re/1 -> U_ctl_calc19/7(Uni_re)
  Uc_im/1 -> U_ctl_calc19/6(Uc_im)
  Uc_re/1 -> U_ctl_calc19/5(Uc_re)
  Ub_im/1 -> U_ctl_calc19/4(Ub_im)
  Ub_re/1 -> U_ctl_calc19/3(Ub_re)
  Ua_im/1 -> U_ctl_calc19/2(Ua_im)
  Ua_re/1 -> U_ctl_calc19/1(Ua_re)
  U_ctl_calc19/14(dc_ph) -> U_ctl_logic19/14(dc_ph)
  U_ctl_calc19/13(db_ph) -> U_ctl_logic19/13(db_ph)
  U_ctl_calc19/12(da_ph) -> U_ctl_logic19/12(da_ph)
  U_ctl_calc19/11(tr_all_non_zero) -> U_ctl_logic19/11(tr_all_non_zero)
  U_ctl_calc19/10(zv_all_non_zero) -> U_ctl_logic19/10(zv_all_non_zero)
  U_ctl_calc19/9(dc_eq_da) -> U_ctl_logic19/9(dc_eq_da)
  U_ctl_calc19/8(db_eq_dc) -> U_ctl_logic19/8(db_eq_dc)
  U_ctl_calc19/7(da_eq_db) -> U_ctl_logic19/7(da_eq_db)
  U_ctl_calc19/6(Y_if) -> U_ctl_logic19/6(Y_if)
  U_ctl_calc19/5(Y_fk) -> U_ctl_logic19/5(Y_fk)
  U_ctl_calc19/4(Y_ni) -> U_ctl_logic19/4(Y_ni)
  U_ctl_calc19/3(Y_c) -> U_ctl_logic19/3(Y_c)
  U_ctl_calc19/2(Y_b) -> U_ctl_logic19/2(Y_b)
  U_ctl_calc19/1(Y_a) -> U_ctl_logic19/1(Y_a)
  auto_zv/1 -> 5/1
  auto_tr/1 -> 5/2
  7/1 -> 6/2
  5/1 -> 3/2, 7/1
  1/1 -> 6/1

== system mylib/262_tnznp_line_st_v1 ==
  fast1_time : Inport
  fast2_time : Inport  Port=2
  fast3_time : Inport  Port=3
  fast4_time : Inport  Port=4
  fast1_zero : Inport  Port=5
  fast2_zero : Inport  Port=6
  fast3_zero : Inport  Port=7
  fast4_zero : Inport  Port=8
  block1 : Inport  Port=9
  block2 : Inport  Port=10
  block3 : Inport  Port=11
  block4 : Inport  Port=12
  no_dir1 : Inport  Port=13
  no_dir2 : Inport  Port=14
  no_dir3 : Inport  Port=15
  no_dir4 : Inport  Port=16
  dir_to_line : Inport  Port=17
  Ia_re : Inport  Port=18
  Ia_im : Inport  Port=19
  Ib_re : Inport  Port=20
  Ib_im : Inport  Port=21
  Ic_re : Inport  Port=22
  Ic_im : Inport  Port=23
  I0_re : Inport  Port=24
  I0_im : Inport  Port=25
  jmp_a : Inport  Port=26
  jmp_b : Inport  Port=27
  jmp_c : Inport  Port=28
  {1..3,33} (4 alike) : Logic  Operator=OR  Inputs=4  AllPortsSameDT=off  OutDataTypeStr=boolean
  200_det18_ph : Subsystem  mask{det=[0, Iph_max, 0, 0]}
      mask prompts: det "det [max_min, set, dir_to_line, dir_to_bus]"
      mask init:
      | max_min = det(1);
      | set = det(2);
      | dir_to_line = det(3);
      | dir_to_bus = det(4);
  218_det18 : Subsystem  mask{det=[0, I0_max, dir_to_line, dir_to_bus]}
      mask prompts: det "det [max_min, set, dir_to_line, dir_to_bus]"
      mask init:
      | max_min = det(1);
      | set = det(2);
      | dir_to_line = det(3);
      | dir_to_bus = det(4);
  230_st18_ph : Subsystem  AncestorBlock=mylib/230_st18_ph  mask{st18_ph=[only_K1, only_K2, only_K3, jmp_in_zone, T_reset, T_fast, T_st, T_out]}
      mask prompts: st18_ph "st18_ph [only_K1, only_K2, only_K3, jmp_in_zone, T_reset, T_fast, T_st, T_out]"
      mask init:
      | only_K1 = st18_ph(1);
      | only_K2 = st18_ph(2); 
      | only_K3 = st18_ph(3); 
      | jmp_in_zone = st18_ph(4);
      | T_reset = st18_ph(5);
      | T_fast = st18_ph(6); 
      | T_st = st18_ph(7); 
      | T_out = st18_ph(8);
  Constant : Constant
  Constant10 : Constant  Value=0
  Constant11 : Constant  Value=0
  Constant12 : Constant
  Constant13 : Constant  Value=0
  Constant3 : Constant  Value=I0_calc
  Switch : Switch  Criteria=u2 > Threshold
  Switch1 : Switch  Criteria=u2 > Threshold
  simpcomp : $bdroot/simpcomp  SystemSampleTime=-1  Latency=0  AutoFrameSizeCalculation=off
  avar : Outport
  avar1 : Outport  Port=2
  Y : Outport  Port=3
  Y_a : Outport  Port=4
  Y_b : Outport  Port=5
  Y_c : Outport  Port=6
  fast : Outport  Port=7
  fast_a : Outport  Port=8
  fast_b : Outport  Port=9
  fast_c : Outport  Port=10
  wires:
  Constant13/1 -> 200_det18_ph/2(start2), 200_det18_ph/3(start3), 200_det18_ph/4(start4), 200_det18_ph/6(block2), 200_det18_ph/7(block3), 200_det18_ph/11(no_dir3), 200_det18_ph/12(no_dir4), 200_det18_ph/13(block_a), 200_det18_ph/14(block_b), 200_det18_ph/15(block_c), 200_det18_ph/22(dir_to_line_a), 200_det18_ph/23(dir_to_line_b), 200_det18_ph/24(dir_to_line_c), 200_det18_ph/10(no_dir2), 200_det18_ph/8(block4)
  Constant12/1 -> 200_det18_ph/9(no_dir1)
  1/1 -> 230_st18_ph/3(fast1_zero)
  33/1 -> 230_st18_ph/1(fast1_time)
  218_det18/2(Y) -> 200_det18_ph/1(start1)
  jmp_c/1 -> 230_st18_ph/17(jmp_c)
  jmp_b/1 -> 230_st18_ph/16(jmp_b)
  jmp_a/1 -> 230_st18_ph/15(jmp_a)
  Constant11/1 -> 230_st18_ph/2(fast2_time), 230_st18_ph/4(fast2_zero), 230_st18_ph/6(block2), 230_st18_ph/7(block3), 230_st18_ph/8(block4), 230_st18_ph/12(alt_in_a), 230_st18_ph/13(alt_in_b), 230_st18_ph/14(alt_in_c)
  200_det18_ph/5(Y_c) -> 230_st18_ph/11(in_c)
  200_det18_ph/4(Y_b) -> 230_st18_ph/10(in_b)
  200_det18_ph/3(Y_a) -> 230_st18_ph/9(in_a)
  230_st18_ph/6(fast) -> fast/1
  230_st18_ph/7(fast_a) -> fast_a/1
  230_st18_ph/8(fast_b) -> fast_b/1
  230_st18_ph/9(fast_c) -> fast_c/1
  230_st18_ph/5(Y_c) -> Y_c/1
  230_st18_ph/4(Y_b) -> Y_b/1
  230_st18_ph/3(Y_a) -> Y_a/1
  230_st18_ph/2(Y) -> Y/1
  230_st18_ph/1(avar) -> avar1/1
  2/1 -> 230_st18_ph/5(block1), 200_det18_ph/5(block1), 218_det18/5(block1)
  3/1 -> 218_det18/9(no_dir1)
  Constant10/1 -> 218_det18/2(start2), 218_det18/3(start3), 218_det18/4(start4), 218_det18/6(block2), 218_det18/7(block3), 218_det18/8(block4), 218_det18/10(no_dir2), 218_det18/11(no_dir3), 218_det18/12(no_dir4)
  Constant/1 -> 218_det18/1(start1)
  dir_to_line/1 -> 218_det18/15(dir_to_line)
  Switch1/1 -> 218_det18/14(in_im)
  Switch/1 -> 218_det18/13(in_re)
  simpcomp/2 -> Switch1/1
  I0_im/1 -> Switch1/3
  simpcomp/1 -> Switch/1
  I0_re/1 -> Switch/3
  Constant3/1 -> Switch1/2, Switch/2
  Ic_im/1 -> simpcomp/6, 200_det18_ph/21(in_c_im)
  Ic_re/1 -> simpcomp/5, 200_det18_ph/20(in_c_re)
  Ib_im/1 -> simpcomp/4, 200_det18_ph/19(in_b_im)
  Ib_re/1 -> simpcomp/3, 200_det18_ph/18(in_b_re)
  Ia_im/1 -> simpcomp/2, 200_det18_ph/17(in_a_im)
  Ia_re/1 -> simpcomp/1, 200_det18_ph/16(in_a_re)
  no_dir1/1 -> 3/1
  no_dir3/1 -> 3/3
  no_dir4/1 -> 3/4
  no_dir2/1 -> 3/2
  fast1_time/1 -> 33/1
  fast2_time/1 -> 33/2
  fast3_time/1 -> 33/3
  fast4_time/1 -> 33/4
  fast1_zero/1 -> 1/1
  fast2_zero/1 -> 1/2
  fast3_zero/1 -> 1/3
  fast4_zero/1 -> 1/4
  block1/1 -> 2/1
  block2/1 -> 2/2
  block3/1 -> 2/3
  block4/1 -> 2/4
  218_det18/1(avar) -> avar/1
